simulink model "conSys_3robots_1_vR2014a"  (Simulink 8.3)
settings: Solver=ode3  StartTime=0.0  StopTime=200  FixedStep=Ts  RelTol=1e-3
values from neighbouring files (symbols this model uses):
  ck = double(max(abs([par.q0_r1;par.q0_r2] - [par.q0r_r1;par.q0r_r2]))*20/7000 + 6)    [startUp_conSys_2robots_1_vGPU_vR2014a.m]    (also in startUp_conSys_2robots_1_vR2014a.m = max(abs([par.q0_r1;par.q0_r2] - [par.q0r_r1;par.q0r_r2]))*20; startUp_conSys_2robots_2_vR2014a.m = max(abs([par.q0_r1;par.q0_r2] - [par.q0r_r1;par.q0r_r2]))*20; startUp_conSys_2robots_3_vR2014a.m = max(abs([par.q0_r1;par.q0_r2] - [par.q0r_r1;par.q0r_r2]))*20; startUp_conSys_2robots_4_vR2014a.m = max(abs([par.q0_r1;par.q0_r2] - [par.q0r_r1;par.q0r_r2]))*20)
  d0t = dt*ht    (= 0.328)    [startUp_conSys_2robots_1_vGPU_vR2014a.m]    (also in startUp_conSys_2robots_1_vR2014a.m; startUp_conSys_2robots_2_vR2014a.m; startUp_conSys_2robots_3_vR2014a.m; startUp_conSys_2robots_4_vR2014a.m)
  dt = rt*ht    (= 16.4)    [startUp_conSys_2robots_1_vGPU_vR2014a.m]    (also in startUp_conSys_2robots_1_vR2014a.m; startUp_conSys_2robots_2_vR2014a.m; startUp_conSys_2robots_3_vR2014a.m; startUp_conSys_2robots_4_vR2014a.m)
  dx1r_0 = dxc_0 + sin(thc_0)*dd_0 + d_0*cos(thc_0)*dthc_0    [startUp_conSys_2robots_1_vGPU_vR2014a.m]    (also in startUp_conSys_2robots_1_vR2014a.m; startUp_conSys_2robots_2_vR2014a.m; startUp_conSys_2robots_3_vR2014a.m; startUp_conSys_2robots_4_vR2014a.m)
  dx2r_0 = dxc_0 - sin(thc_0)*dd_0 - d_0*cos(thc_0)*dthc_0    [startUp_conSys_2robots_1_vGPU_vR2014a.m]    (also in startUp_conSys_2robots_1_vR2014a.m; startUp_conSys_2robots_2_vR2014a.m; startUp_conSys_2robots_3_vR2014a.m; startUp_conSys_2robots_4_vR2014a.m)
  dy1r_0 = dyc_0 + cos(thc_0)*dd_0 - d_0*sin(thc_0)*dthc_0    [startUp_conSys_2robots_1_vGPU_vR2014a.m]    (also in startUp_conSys_2robots_1_vR2014a.m; startUp_conSys_2robots_2_vR2014a.m; startUp_conSys_2robots_3_vR2014a.m; startUp_conSys_2robots_4_vR2014a.m)
  dy2r_0 = dyc_0 - cos(thc_0)*dd_0 + d_0*sin(thc_0)*dthc_0    [startUp_conSys_2robots_1_vGPU_vR2014a.m]    (also in startUp_conSys_2robots_1_vR2014a.m; startUp_conSys_2robots_2_vR2014a.m; startUp_conSys_2robots_3_vR2014a.m; startUp_conSys_2robots_4_vR2014a.m)
  ht = .02    (= 0.02)    [startUp_conSys_2robots_1_vGPU_vR2014a.m]    (also in startUp_conSys_2robots_1_vR2014a.m; startUp_conSys_2robots_2_vR2014a.m; startUp_conSys_2robots_3_vR2014a.m; startUp_conSys_2robots_4_vR2014a.m)
  rt = 820    [startUp_conSys_2robots_1_vGPU_vR2014a.m]    (also in startUp_conSys_2robots_1_vR2014a.m; startUp_conSys_2robots_2_vR2014a.m; startUp_conSys_2robots_3_vR2014a.m; startUp_conSys_2robots_4_vR2014a.m)
  TD = ss(Atd,Btd,Ctd,Dtd,Ts)    [startUp_conSys_2robots_1_vGPU_vR2014a.m]    (also in startUp_conSys_2robots_1_vR2014a.m; startUp_conSys_2robots_2_vR2014a.m; startUp_conSys_2robots_3_vR2014a.m; startUp_conSys_2robots_4_vR2014a.m)
  Ts = 1/200    (= 0.005)    [startUp_conSys_2robots_1_vGPU_vR2014a.m]    (also in startUp_conSys_2robots_1_vR2014a.m = 0.0125; startUp_conSys_2robots_2_vR2014a.m = 0.01; startUp_conSys_2robots_3_vR2014a.m; startUp_conSys_2robots_4_vR2014a.m)
undefined symbols (not defined in the file or in its folder): Beta_Correction_1b, Beta_Correction_2b, Beta_Correction_3b, Beta_Correction_4b, DiscIntNeverNeededParam, dth1r_0, dth2r_0, dth3r_0, dx3r_0, dy3r_0, par, th1r_0, th2r_0, th3r_0, x1r_0, x2r_0, x3r_0, y1r_0, y2r_0, y3r_0
undefined symbols (not defined in the file): ADAMS_cwd, ADAMS_exec, ADAMS_host, ADAMS_init, ADAMS_inputs, ADAMS_outputs, ADAMS_prefix, ADAMS_static, ADAMS_sysdir
libraries: simulink x26, cstblocks x11
(part 2 of 3)

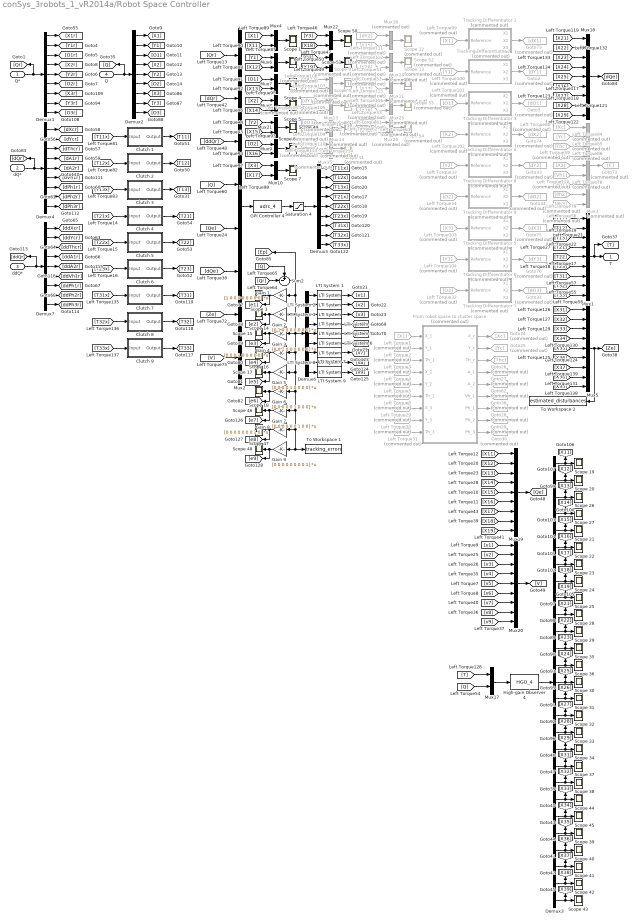
== system conSys_3robots_1_vR2014a/Robot Space Controller ==
  Q* : Inport
  dQ* : Inport  Port=2
  ddQ* : Inport  Port=3
  Q : Inport  Port=4
  Clutch 1 : Subsystem
  Clutch 2 : Subsystem
  Clutch 3 : Subsystem
  Clutch 4 : Subsystem
  Clutch 5 : Subsystem
  Clutch 6 : Subsystem
  Clutch 7 : Subsystem
  Clutch 8 : Subsystem
  Clutch 9 : Subsystem
  Demux{1..2,4..7} (6 alike) : Demux  Outputs=9
  Demux3 : Demux  Outputs=27
  From robot space to cluster space : Subsystem  Commented=on
  GPI Controller 4 : S-Function  FunctionName=adrc_4  Parameters=par  EnableBusSupport=off
  Gain 1 : Gain  Gain=[1 0 0 0 0 0 0 0 0]  Multiplication=Matrix(K*u)
  Gain 2 : Gain  Gain=[0 1 0 0 0 0 0 0 0]  Multiplication=Matrix(K*u)
  Gain 3 : Gain  Gain=[0 0 1 0 0 0 0 0 0]  Multiplication=Matrix(K*u)
  Gain 4 : Gain  Gain=[0 0 0 1 0 0 0 0 0]  Multiplication=Matrix(K*u)
  Gain 5 : Gain  Gain=[0 0 0 0 1 0 0 0 0]  Multiplication=Matrix(K*u)
  Gain 6 : Gain  Gain=[0 0 0 0 0 1 0 0 0]  Multiplication=Matrix(K*u)
  Gain 7 : Gain  Gain=[0 0 0 0 0 0 1 0 0]  Multiplication=Matrix(K*u)
  Gain 8 : Gain  Gain=[0 0 0 0 0 0 0 1 0]  Multiplication=Matrix(K*u)
  Gain 9 : Gain  Gain=[0 0 0 0 0 0 0 0 1]  Multiplication=Matrix(K*u)
  Goto2 : Goto  Commented=on  GotoTag=dY1
  Goto24 : Goto  Commented=on  GotoTag=Xc
  Goto25 : Goto  Commented=on  GotoTag=Yc
  Goto26 : Goto  Commented=on  GotoTag=Thc
  Goto27 : Goto  Commented=on  GotoTag=A1
  Goto28 : Goto  Commented=on  GotoTag=Ph1
  Goto29 : Goto  Commented=on  GotoTag=Ph2
  Goto3 : Goto  Commented=on  GotoTag=dO1
  Goto30 : Goto  Commented=on  GotoTag=Ph3
  Goto32 : Goto  Commented=on  GotoTag=dO3
  Goto33 : Goto  Commented=on  GotoTag=dY2
  Goto34 : Goto  Commented=on  GotoTag=dO2
  Goto36 : Goto  Commented=on  GotoTag=Vh1
  Goto62 : Goto  Commented=on  GotoTag=A2
  Goto72 : Goto  Commented=on  GotoTag=C
  Goto73 : Goto  Commented=on  GotoTag=dX1
  Goto74 : Goto  Commented=on  GotoTag=dX2
  Goto75 : Goto  Commented=on  GotoTag=dX3
  Goto76 : Goto  Commented=on  GotoTag=dY3
  High-gain Observer 4 : S-Function  FunctionName=HGO_4  Parameters=par  EnableBusSupport=off
  LTI System {1..2,4..5,7..8} (6 alike) : cstblocks/LTI System  sys=par.Gz_1  IC=[]
  LTI System 3 : cstblocks/LTI System  sys=par.Gz_2  IC=[]
  LTI System 6 : cstblocks/LTI System  sys=par.Gz_2  IC=[]
  LTI System 9 : cstblocks/LTI System  sys=par.Gz_2  IC=[]
  Left Torque1 : From  Commented=on  GotoTag=X1
  Left Torque100 : From  Commented=on  GotoTag=Y1
  Left Torque101 : From  Commented=on  GotoTag=O1
  Left Torque102 : From  Commented=on  GotoTag=X2
  Left Torque103 : From  Commented=on  GotoTag=X3
  Left Torque104 : From  Commented=on  GotoTag=Y3
  Left Torque105 : From  Commented=on  GotoTag=dY1
  Left Torque106 : From  Commented=on  GotoTag=X22
  Left Torque107 : From  Commented=on  GotoTag=dX1
  Left Torque108 : From  Commented=on  GotoTag=X21
  Left Torque109 : From  Commented=on  GotoTag=dO1
  Left Torque110 : From  Commented=on  GotoTag=X23
  Left Torque111 : From  Commented=on  GotoTag=dY2
  Left Torque112 : From  Commented=on  GotoTag=X25
  Left Torque113 : From  Commented=on  GotoTag=dX2
  Left Torque114 : From  Commented=on  GotoTag=X24
  Left Torque115 : From  Commented=on  GotoTag=dX3
  Left Torque116 : From  Commented=on  GotoTag=X27
  Left Torque120 : From  Commented=on  GotoTag=Vh1
  Left Torque2 : From  Commented=on  GotoTag=Y1
  Left Torque29 : From  Commented=on  GotoTag=X3
  Left Torque3 : From  Commented=on  GotoTag=O1
  Left Torque30 : From  Commented=on  GotoTag=Y3
  Left Torque31 : From  Commented=on  GotoTag=O3
  Left Torque32 : From  Commented=on  GotoTag=O3
  Left Torque33 : From  Commented=on  GotoTag=Y2
  Left Torque34 : From  Commented=on  GotoTag=O2
  Left Torque4 : From  Commented=on  GotoTag=X2
  Left Torque5 : From  Commented=on  GotoTag=Y2
  Left Torque51 : From  Commented=on  GotoTag=dO2
  Left Torque52 : From  Commented=on  GotoTag=X26
  Left Torque53 : From  Commented=on  GotoTag=dY3
  Left Torque58 : From  Commented=on  GotoTag=Ph3
  Left Torque59 : From  Commented=on  GotoTag=A2
  Left Torque6 : From  Commented=on  GotoTag=O2
  Left Torque61 : From  Commented=on  GotoTag=X28
  Left Torque62 : From  Commented=on  GotoTag=dO3
  Left Torque63 : From  Commented=on  GotoTag=X29
  Left Torque78 : From  Commented=on  GotoTag=Ph1
  Left Torque79 : From  Commented=on  GotoTag=Ph2
  Left Torque80 : From  Commented=on  GotoTag=Xc
  Left Torque84 : From  Commented=on  GotoTag=Yc
  Left Torque85 : From  Commented=on  GotoTag=Thc
  Left Torque86 : From  Commented=on  GotoTag=A1
  Left Torque99 : From  Commented=on  GotoTag=X1
  Mux{1,5,18..20} (5 alike) : Mux  Inputs=9
  Mux{4,6..10,17,21..23} (10 alike) : Mux  Inputs=2
  Mux{11..16,24..26} (9 alike) : Mux  Commented=on  Inputs=2
  Mux2 : Mux  Inputs=8
  Mux3 : Mux  Commented=on  Inputs=9
  Saturation 4 : Saturate  UpperLimit=100  LowerLimit=-100
  Scope {1..7,14..51} (45 alike) : Scope
      Scope 1 settings: YMin=-2000  YMax=16000  SaveName=ScopeData37
      Scope 14 settings: YMin=-100  YMax=2000  SaveName=ScopeData77
      Scope 15 settings: YMin=-1  YMax=4  SaveName=ScopeData78
      Scope 16 settings: YMin=-100  YMax=2000  SaveName=ScopeData82
      Scope 17 settings: YMin=-100  YMax=2000  SaveName=ScopeData83
      Scope 18 settings: YMin=-1  YMax=4  SaveName=ScopeData84
      Scope 19 settings: YMin=-2000  YMax=16000  SaveName=ScopeData86
      Scope 2 settings: YMin=-2000  YMax=16000  SaveName=ScopeData39
      Scope 20 settings: YMin=0  YMax=10000  SaveName=ScopeData87
      Scope 21 settings: YMin=0  YMax=5000  SaveName=ScopeData88
      Scope 22 settings: SaveName=ScopeData90
      Scope 23 settings: YMin=-10  YMax=100  SaveName=ScopeData91
      Scope 24 settings: YMin=-50  YMax=50  SaveName=ScopeData92
      Scope 25 settings: YMin=-6  YMax=6  SaveName=ScopeData93
      Scope 26 settings: SaveName=ScopeData94
      Scope 27 settings: TimeRange=388  YMin=-6  YMax=60  SaveName=ScopeData95
      Scope 28 settings: YMin=0  YMax=10000  SaveName=ScopeData96
      Scope 29 settings: YMin=0  YMax=10000  SaveName=ScopeData97
      Scope 3 settings: YMin=-100  YMax=2000  SaveName=ScopeData40
      Scope 30 settings: YMin=-50  YMax=50  SaveName=ScopeData98
      Scope 31 settings: YMin=-1  YMax=1  SaveName=ScopeData99
      Scope 32 settings: YMin=-60  YMax=60  SaveName=ScopeData100
      Scope 33 settings: YMin=-1  YMax=1  SaveName=ScopeData101
      Scope 34 settings: YMin=-1  YMax=1  SaveName=ScopeData102
      Scope 35 settings: SaveName=ScopeData103
      Scope 36 settings: YMin=-60  YMax=60  SaveName=ScopeData104
      Scope 37 settings: YMin=-600  YMax=600  SaveName=ScopeData26
      Scope 38 settings: YMin=-600  YMax=600  SaveName=ScopeData27
      Scope 39 settings: YMin=-600  YMax=600  SaveName=ScopeData28
      Scope 4 settings: YMin=-2000  YMax=16000  SaveName=ScopeData41
      Scope 40 settings: YMin=-1  YMax=1  SaveName=ScopeData42
      Scope 41 settings: YMin=-600  YMax=600  SaveName=ScopeData52
      Scope 42 settings: YMin=-600  YMax=600  SaveName=ScopeData53
      Scope 43 settings: YMin=-1  YMax=1  SaveName=ScopeData54
      Scope 44 settings: SaveName=ScopeData55
      Scope 45 settings: YMin=-600  YMax=600  SaveName=ScopeData56
      Scope 46 settings: YMin=-100  YMax=2000  SaveName=ScopeData57
      Scope 47 settings: YMin=-100  YMax=2000  SaveName=ScopeData58
      Scope 48 settings: YMin=-1  YMax=4  SaveName=ScopeData59
      Scope 49 settings: YMin=-2000  YMax=16000  SaveName=ScopeData60
      Scope 5 settings: YMin=-2000  YMax=16000  SaveName=ScopeData43
      Scope 50 settings: YMin=-20  YMax=20  SaveName=ScopeData62
      Scope 51 settings: YMin=-20  YMax=20  SaveName=ScopeData63
      Scope 6 settings: YMin=-20  YMax=20  SaveName=ScopeData44
      Scope 7 settings: YMin=-20  YMax=20  SaveName=ScopeData45
  Scope {8..13,52..54} (9 alike) : Scope  Commented=on
      Scope 10 settings: YMin=-2  YMax=2  SaveName=ScopeData46
      Scope 11 settings: YMin=-40  YMax=40  SaveName=ScopeData47
      Scope 12 settings: YMin=-2  YMax=2  SaveName=ScopeData73
      Scope 13 settings: YMin=-2  YMax=2  SaveName=ScopeData74
      Scope 52 settings: YMin=-2  YMax=2  SaveName=ScopeData64
      Scope 53 settings: YMin=-2  YMax=2  SaveName=ScopeData65
      Scope 54 settings: YMin=-2  YMax=2  SaveName=ScopeData66
      Scope 8 settings: YMin=-2000  YMax=16000  SaveName=ScopeData75
      Scope 9 settings: YMin=-2000  YMax=2000  SaveName=ScopeData76
  Sum2 : Sum  Inputs=+-|
  To Workspace 1 : ToWorkspace  VariableName=tracking_errors  SaveFormat=Structure With Time  SampleTime=-1
  To Workspace 2 : ToWorkspace  VariableName=estimated_disturbances  SaveFormat=Structure With Time  SampleTime=-1
  Tracking Differentiator 1 : Subsystem  Commented=on
  Tracking Differentiator 2 : Subsystem  Commented=on
  Tracking Differentiator 3 : Subsystem  Commented=on
  Tracking Differentiator 4 : Subsystem  Commented=on
  Tracking Differentiator 5 : Subsystem  Commented=on
  Tracking Differentiator 6 : Subsystem  Commented=on
  Tracking Differentiator 7 : Subsystem  Commented=on
  Tracking Differentiator 8 : Subsystem  Commented=on
  Tracking Differentiator 9 : Subsystem  Commented=on
  T : Outport
  wires:
  From robot space to cluster space/5(A_2) -> Goto62/1
  From robot space to cluster space/8(Ph_2) -> Goto29/1
  From robot space to cluster space/7(Ph_1) -> Goto28/1
  From robot space to cluster space/3(Th_c) -> Goto26/1
  From robot space to cluster space/2(Y_c) -> Goto25/1
  From robot space to cluster space/1(X_c) -> Goto24/1
  Q/1 -> Demux2/1, [Q]
  Demux2/1 -> [X1]
  Demux2/2 -> [Y1]
  Demux2/3 -> [O1]
  Demux2/4 -> [X2]
  Demux2/5 -> [Y2]
  Demux2/6 -> [O2]
  Left Torque1/1 -> From robot space to cluster space/1(X_1)
  Left Torque2/1 -> From robot space to cluster space/2(Y_1)
  Left Torque3/1 -> From robot space to cluster space/3(Th_1)
  Left Torque4/1 -> From robot space to cluster space/4(X_2)
  Left Torque5/1 -> From robot space to cluster space/5(Y_2)
  Left Torque6/1 -> From robot space to cluster space/6(Th_2)
  Mux2/1 -> GPI Controller 4/1
  Demux5/1 -> [T11x]
  Demux5/2 -> [T12x]
  Demux5/3 -> [T13x]
  GPI Controller 4/1 -> Saturation 4/1
  Saturation 4/1 -> Demux5/1
  Demux5/4 -> [T21x]
  Demux5/5 -> [T22x]
  Demux5/6 -> [T23x]
  [Qr] -> Sum2/2
  [Q] -> Sum2/1
  Demux6/1 -> LTI System 1/1
  Demux6/2 -> LTI System 2/1
  Demux6/3 -> LTI System 3/1
  [T11x] -> Clutch 1/1(Input)
  Clutch 1/1(Output) -> [T11]
  [T12x] -> Clutch 2/1(Input)
  Clutch 2/1(Output) -> [T12]
  [T13x] -> Clutch 3/1(Input)
  Clutch 3/1(Output) -> [T13]
  [T21x] -> Clutch 4/1(Input)
  Clutch 4/1(Output) -> [T21]
  [T22x] -> Clutch 5/1(Input)
  Clutch 5/1(Output) -> [T22]
  [T23x] -> Clutch 6/1(Input)
  Clutch 6/1(Output) -> [T23]
  [T11] -> Mux1/1
  [T23] -> Mux1/6
  [T21] -> Mux1/4
  [T22] -> Mux1/5
  [T12] -> Mux1/2
  [T13] -> Mux1/3
  Mux1/1 -> [T], T/1
  Q*/1 -> [Qr], Demux1/1
  Demux1/1 -> [X1r]
  Demux1/2 -> [Y1r]
  Demux1/3 -> [O1r]
  Demux1/4 -> [X2r]
  Demux1/5 -> [Y2r]
  Demux1/6 -> [O2r]
  dQ*/1 -> [dQr], Demux4/1
  Demux4/1 -> [dXcr]
  Demux4/2 -> [dYcr]
  Demux4/3 -> [dThcr]
  Demux4/4 -> [dA1r]
  Demux7/1 -> [ddXcr]
  Demux7/2 -> [ddYcr]
  Demux7/3 -> [ddThcr]
  Demux7/4 -> [ddA1r]
  ddQ*/1 -> [ddQr], Demux7/1
  Demux6/4 -> LTI System 4/1
  Demux6/5 -> LTI System 5/1
  Demux6/6 -> LTI System 6/1
  [Qr] -> Mux2/1
  [ddQr] -> Mux2/3
  [Q] -> Mux2/4
  [Ze] -> Mux2/7
  [Qe] -> Mux2/5
  [dQe] -> Mux2/6
  [V] -> Mux2/8
  Left Torque80/1 -> Mux3/1
  Left Torque86/1 -> Mux3/4
  Left Torque84/1 -> Mux3/2
  Left Torque85/1 -> Mux3/3
  Mux3/1 -> Goto72/1
  [X11] -> Mux4/2
  [X1] -> Mux4/1
  Mux4/1 -> Scope 1/1
  [X12] -> Mux6/2
  [Y1] -> Mux6/1
  Mux6/1 -> Scope 2/1
  [X13] -> Mux7/2
  [O1] -> Mux7/1
  Mux7/1 -> Scope 4/1
  [X14] -> Mux8/2
  [X2] -> Mux8/1
  Mux8/1 -> Scope 5/1
  [X16] -> Mux9/2
  [O2] -> Mux9/1
  Mux9/1 -> Scope 6/1
  [X17] -> Mux10/2
  [X3] -> Mux10/1
  Mux10/1 -> Scope 7/1
  Left Torque99/1 -> Tracking Differentiator 1/1(Reference)
  Left Torque100/1 -> Tracking Differentiator 2/1(Reference)
  Left Torque101/1 -> Tracking Differentiator 3/1(Reference)
  Left Torque102/1 -> Tracking Differentiator 4/1(Reference)
  Left Torque103/1 -> Tracking Differentiator 5/1(Reference)
  Left Torque104/1 -> Tracking Differentiator 6/1(Reference)
  Tracking Differentiator 1/2(X2) -> Goto73/1
  Tracking Differentiator 2/2(X2) -> Goto2/1
  Tracking Differentiator 3/2(X2) -> Goto3/1
  Tracking Differentiator 4/2(X2) -> Goto74/1
  Tracking Differentiator 5/2(X2) -> Goto75/1
  Tracking Differentiator 6/2(X2) -> Goto76/1
  Left Torque108/1 -> Mux12/2
  Left Torque107/1 -> Mux12/1
  Mux12/1 -> Scope 8/1
  Left Torque106/1 -> Mux13/2
  Left Torque105/1 -> Mux13/1
  Mux13/1 -> Scope 9/1
  Left Torque110/1 -> Mux14/2
  Left Torque109/1 -> Mux14/1
  Mux14/1 -> Scope 10/1
  Left Torque114/1 -> Mux15/2
  Left Torque113/1 -> Mux15/1
  Mux15/1 -> Scope 11/1
  Left Torque112/1 -> Mux16/2
  Left Torque111/1 -> Mux16/1
  Mux16/1 -> Scope 12/1
  Left Torque116/1 -> Mux11/2
  Left Torque115/1 -> Mux11/1
  Mux11/1 -> Scope 13/1
  LTI System 1/1 -> [v1]
  LTI System 2/1 -> [v2]
  LTI System 3/1 -> [v3]
  LTI System 4/1 -> [v4]
  LTI System 5/1 -> [v5]
  LTI System 6/1 -> [v6]
  Gain 1/1 -> [e1], Scope 3/1
  Gain 2/1 -> [e2], Scope 14/1
  Gain 3/1 -> [e3], Scope 15/1
  Gain 4/1 -> [e4], Scope 16/1
  Gain 5/1 -> [e5], Scope 17/1
  Gain 6/1 -> [e6], Scope 18/1
  Mux17/1 -> High-gain Observer 4/1
  Demux3/9 -> Scope 25/1, [X19]
  Demux3/7 -> [X17], Scope 23/1
  Demux3/8 -> [X18], Scope 24/1
  Demux3/5 -> [X15], Scope 21/1
  Demux3/6 -> [X16], Scope 22/1
  High-gain Observer 4/1 -> Demux3/1
  Demux3/3 -> Scope 26/1, [X13]
  Demux3/4 -> Scope 27/1, [X14]
  Demux3/1 -> Scope 19/1, [X11]
  Demux3/2 -> Scope 20/1, [X12]
  Demux3/17 -> Scope 33/1, [X28]
  Demux3/13 -> [X24], Scope 36/1
  Demux3/12 -> [X23], Scope 35/1
  Demux3/18 -> [X29], Scope 34/1
  Demux3/15 -> Scope 31/1, [X26]
  Demux3/10 -> [X21], Scope 28/1
  Demux3/11 -> [X22], Scope 29/1
  Demux3/16 -> Scope 32/1, [X27]
  Demux3/14 -> Scope 30/1, [X25]
  [X21] -> Mux18/1
  [X26] -> Mux18/6
  [X24] -> Mux18/4
  [X25] -> Mux18/5
  [X22] -> Mux18/2
  [X23] -> Mux18/3
  Mux18/1 -> [dQe]
  Demux2/7 -> [X3]
  Demux2/8 -> [Y3]
  Demux2/9 -> [O3]
  Demux1/7 -> [X3r]
  Demux1/8 -> [Y3r]
  Demux1/9 -> [O3r]
  Demux4/7 -> [dPh1r]
  Demux4/8 -> [dPh2r]
  Demux4/5 -> [dA2r]
  Demux4/6 -> [dVh1r]
  Demux4/9 -> [dPh3r]
  Demux7/7 -> [ddPh1r]
  Demux7/8 -> [ddPh2r]
  Demux7/9 -> [ddPh3r]
  Demux7/5 -> [ddA2r]
  Demux7/6 -> [ddVh1r]
  [T31x] -> Clutch 7/1(Input)
  Clutch 7/1(Output) -> [T31]
  [T32x] -> Clutch 8/1(Input)
  Clutch 8/1(Output) -> [T32]
  [T33x] -> Clutch 9/1(Input)
  Clutch 9/1(Output) -> [T33]
  Left Torque29/1 -> From robot space to cluster space/7(X_3)
  Left Torque30/1 -> From robot space to cluster space/8(Y_3)
  Left Torque31/1 -> From robot space to cluster space/9(Th_3)
  From robot space to cluster space/4(A_1) -> Goto27/1
  From robot space to cluster space/6(Vh_1) -> Goto36/1
  From robot space to cluster space/9(Ph_3) -> Goto30/1
  Left Torque32/1 -> Tracking Differentiator 7/1(Reference)
  Tracking Differentiator 7/2(X2) -> Goto32/1
  Left Torque33/1 -> Tracking Differentiator 8/1(Reference)
  Tracking Differentiator 8/2(X2) -> Goto33/1
  Left Torque34/1 -> Tracking Differentiator 9/1(Reference)
  Tracking Differentiator 9/2(X2) -> Goto34/1
  [T] -> Mux17/1
  [Q] -> Mux17/2
  [T33] -> Mux1/9
  [T31] -> Mux1/7
  [T32] -> Mux1/8
  Left Torque59/1 -> Mux3/5
  Left Torque58/1 -> Mux3/9
  Left Torque120/1 -> Mux3/6
  Left Torque78/1 -> Mux3/7
  Left Torque79/1 -> Mux3/8
  [X27] -> Mux18/7
  [X29] -> Mux18/9
  [X28] -> Mux18/8
  [X31] -> Mux5/1
  [X36] -> Mux5/6
  [X34] -> Mux5/4
  [X35] -> Mux5/5
  [X32] -> Mux5/2
  [X33] -> Mux5/3
  Mux5/1 -> To Workspace 2/1, [Ze]
  [X39] -> Mux5/9
  [X37] -> Mux5/7
  [X38] -> Mux5/8
  Demux3/26 -> [X38], Scope 42/1
  Demux3/22 -> Scope 45/1, [X34]
  Demux3/21 -> Scope 44/1, [X33]
  Demux3/27 -> Scope 43/1, [X39]
  Demux3/24 -> [X36], Scope 40/1
  Demux3/19 -> Scope 37/1, [X31]
  Demux3/20 -> Scope 38/1, [X32]
  Demux3/25 -> [X37], Scope 41/1
  Demux3/23 -> [X35], Scope 39/1
  [X11] -> Mux19/1
  [X16] -> Mux19/6
  [X14] -> Mux19/4
  [X15] -> Mux19/5
  [X12] -> Mux19/2
  [X13] -> Mux19/3
  Mux19/1 -> [Qe]
  [X19] -> Mux19/9
  [X17] -> Mux19/7
  [X18] -> Mux19/8
  [v1] -> Mux20/1
  [v6] -> Mux20/6
  [v4] -> Mux20/4
  [v5] -> Mux20/5
  [v2] -> Mux20/2
  [v3] -> Mux20/3
  Mux20/1 -> [V]
  [v9] -> Mux20/9
  [v7] -> Mux20/7
  [v8] -> Mux20/8
  [dQr] -> Mux2/2
  Demux5/7 -> [T31x]
  Demux5/8 -> [T32x]
  Demux5/9 -> [T33x]
  Demux6/7 -> LTI System 7/1
  LTI System 7/1 -> [v7]
  LTI System 8/1 -> [v8]
  LTI System 9/1 -> [v9]
  Demux6/8 -> LTI System 8/1
  Demux6/9 -> LTI System 9/1
  Gain 7/1 -> Scope 46/1, [e7]
  Gain 8/1 -> [e8], Scope 47/1
  Gain 9/1 -> Scope 48/1, [e9]
  [X15] -> Mux21/2
  Mux21/1 -> Scope 49/1
  [Y2] -> Mux21/1
  [X18] -> Mux22/2
  [Y3] -> Mux22/1
  Mux22/1 -> Scope 50/1
  [X19] -> Mux23/2
  [O3] -> Mux23/1
  Mux23/1 -> Scope 51/1
  Left Torque52/1 -> Mux24/2
  Left Torque51/1 -> Mux24/1
  Mux24/1 -> Scope 52/1
  Left Torque61/1 -> Mux25/2
  Left Torque53/1 -> Mux25/1
  Mux25/1 -> Scope 53/1
  Left Torque63/1 -> Mux26/2
  Left Torque62/1 -> Mux26/1
  Mux26/1 -> Scope 54/1
  Sum2/1 -> Demux6/1, To Workspace 1/1, Gain 9/1, Gain 8/1, Gain 7/1, Gain 6/1, Gain 5/1, Gain 4/1, Gain 3/1, Gain 2/1, Gain 1/1, [Ep]

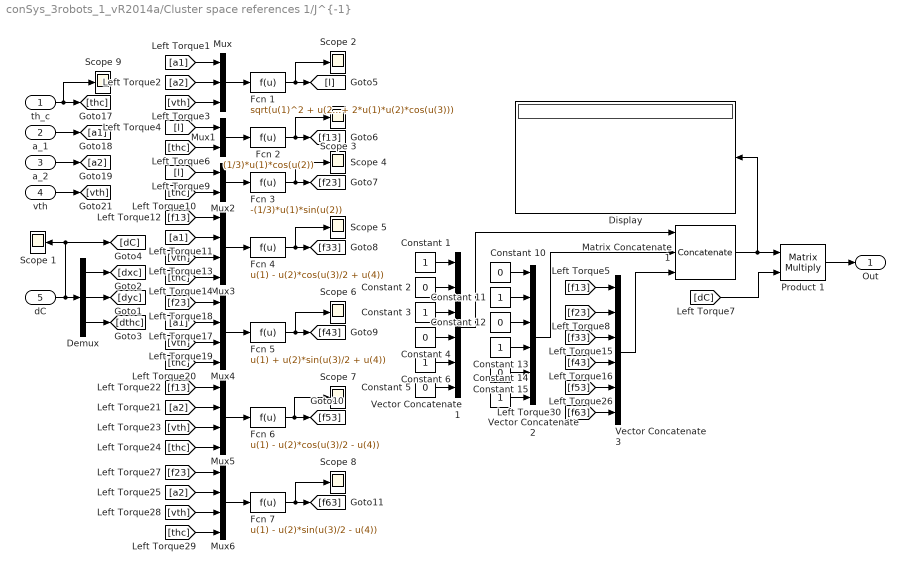
== system conSys_3robots_1_vR2014a/Cluster space references 1/J^{-1} ==
  th_c : Inport
  a_1 : Inport  Port=2
  a_2 : Inport  Port=3
  vth : Inport  Port=4
  dC : Inport  Port=5  PortDimensions=3
  Constant {1,3,6,11,13..14} (6 alike) : Constant
  Constant {2,4..5,10,12,15} (6 alike) : Constant  Value=0
  Demux : Demux  Outputs=3
  Display : Display
  Fcn 1 : Fcn  Expr=sqrt(u(1)^2 + u(2)^2 + 2*u(1)*u(2)*cos(u(3)))
  Fcn 2 : Fcn  Expr=(1/3)*u(1)*cos(u(2))
  Fcn 3 : Fcn  Expr=-(1/3)*u(1)*sin(u(2))
  Fcn 4 : Fcn  Expr=u(1) - u(2)*cos(u(3)/2 + u(4))
  Fcn 5 : Fcn  Expr=u(1) + u(2)*sin(u(3)/2 + u(4))
  Fcn 6 : Fcn  Expr=u(1) - u(2)*cos(u(3)/2 - u(4))
  Fcn 7 : Fcn  Expr=u(1) - u(2)*sin(u(3)/2 - u(4))
  Matrix Concatenate 1 : Concatenate  NumInputs=3  Mode=Multidimensional array  ConcatenateDimension=2
  Mux : Mux  Inputs=3
  Mux1 : Mux  Inputs=2
  Mux2 : Mux  Inputs=2
  Mux{3..6} (4 alike) : Mux
  Product 1 : Product  Multiplication=Matrix(*)
  Scope {1..9} (9 alike) : Scope
      Scope 1 settings: ShowLegends=on  YMin=-500  YMax=500  SaveName=ScopeData33
      Scope 2 settings: ShowLegends=on  YMin=-500  YMax=800  SaveName=ScopeData34
      Scope 3 settings: ShowLegends=on  YMin=-500  YMax=500  SaveName=ScopeData35
      Scope 4 settings: ShowLegends=on  YMin=-500  YMax=500  SaveName=ScopeData36
      Scope 5 settings: ShowLegends=on  YMin=-500  YMax=500  SaveName=ScopeData37
      Scope 6 settings: ShowLegends=on  YMin=-500  YMax=500  SaveName=ScopeData38
      Scope 7 settings: ShowLegends=on  YMin=-500  YMax=500  SaveName=ScopeData39
      Scope 8 settings: ShowLegends=on  YMin=-500  YMax=500  SaveName=ScopeData40
      Scope 9 settings: ShowLegends=on  YMin=-10  YMax=10  SaveName=ScopeData41
  Vector Concatenate 1 : Concatenate  NumInputs=6
  Vector Concatenate 2 : Concatenate  NumInputs=6
  Vector Concatenate 3 : Concatenate  NumInputs=6
  Out : Outport
  wires:
  [f53] -> Vector Concatenate 3/5
  [f43] -> Vector Concatenate 3/4
  [f23] -> Vector Concatenate 3/2
  [f13] -> Vector Concatenate 3/1
  Constant 14/1 -> Vector Concatenate 2/6
  Constant 15/1 -> Vector Concatenate 2/5
  Constant 13/1 -> Vector Concatenate 2/4
  Constant 12/1 -> Vector Concatenate 2/3
  Constant 11/1 -> Vector Concatenate 2/2
  Constant 10/1 -> Vector Concatenate 2/1
  Vector Concatenate 1/1 -> Matrix Concatenate 1/1
  Constant 5/1 -> Vector Concatenate 1/6
  Constant 6/1 -> Vector Concatenate 1/5
  Constant 4/1 -> Vector Concatenate 1/4
  Constant 3/1 -> Vector Concatenate 1/3
  Constant 2/1 -> Vector Concatenate 1/2
  Constant 1/1 -> Vector Concatenate 1/1
  vth/1 -> [vth]
  a_2/1 -> [a2]
  a_1/1 -> [a1]
  th_c/1 -> Scope 9/1, [thc]
  dC/1 -> Scope 1/1, [dC], Demux/1
  Demux/1 -> [dxc]
  Demux/2 -> [dyc]
  Demux/3 -> [dthc]
  [vth] -> Mux/3
  [a1] -> Mux/1
  [a2] -> Mux/2
  Mux/1 -> Fcn 1/1
  Fcn 1/1 -> Scope 2/1, [l]
  [l] -> Mux1/1
  [thc] -> Mux1/2
  Mux1/1 -> Fcn 2/1
  Fcn 2/1 -> Scope 3/1, [f13]
  Vector Concatenate 2/1 -> Matrix Concatenate 1/2
  Vector Concatenate 3/1 -> Matrix Concatenate 1/3
  Matrix Concatenate 1/1 -> Product 1/1, Display/1
  [dC] -> Product 1/2
  Product 1/1 -> Out/1
  [l] -> Mux2/1
  [thc] -> Mux2/2
  Mux2/1 -> Fcn 3/1
  Fcn 3/1 -> Scope 4/1, [f23]
  [f13] -> Mux3/1
  [a1] -> Mux3/2
  Mux3/1 -> Fcn 4/1
  Fcn 4/1 -> Scope 5/1, [f33]
  [vth] -> Mux3/3
  [thc] -> Mux3/4
  [f33] -> Vector Concatenate 3/3
  [f23] -> Mux4/1
  [a1] -> Mux4/2
  Mux4/1 -> Fcn 5/1
  Fcn 5/1 -> Scope 6/1, [f43]
  [vth] -> Mux4/3
  [thc] -> Mux4/4
  [f13] -> Mux5/1
  [a2] -> Mux5/2
  Mux5/1 -> Fcn 6/1
  Fcn 6/1 -> Scope 7/1, [f53]
  [vth] -> Mux5/3
  [thc] -> Mux5/4
  [f23] -> Mux6/1
  [a2] -> Mux6/2
  Mux6/1 -> Fcn 7/1
  Fcn 7/1 -> Scope 8/1, [f63]
  [vth] -> Mux6/3
  [thc] -> Mux6/4
  [f63] -> Vector Concatenate 3/6

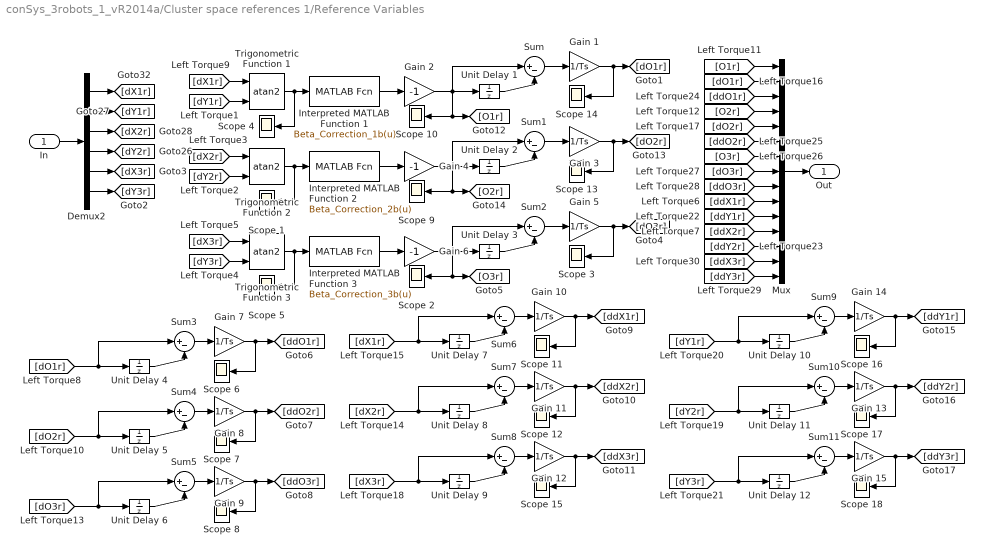
== system conSys_3robots_1_vR2014a/Cluster space references 1/Reference Variables ==
  In : Inport  PortDimensions=6
  Demux2 : Demux  Outputs=6
  Gain {1,3,5,7..15} (12 alike) : Gain  Gain=1/Ts
  Gain 2 : Gain  Gain=-1
  Gain 4 : Gain  Gain=-1
  Gain 6 : Gain  Gain=-1
  Interpreted MATLAB Function 1 : MATLABFcn  MATLABFcn=Beta_Correction_1b(u)  SampleTime=Ts
  Interpreted MATLAB Function 2 : MATLABFcn  MATLABFcn=Beta_Correction_2b(u)  SampleTime=Ts
  Interpreted MATLAB Function 3 : MATLABFcn  MATLABFcn=Beta_Correction_3b(u)  SampleTime=Ts
  Mux : Mux  Inputs=15
  Scope {1..18} (18 alike) : Scope
      Scope 1 settings: YMin=0  YMax=10  SaveName=ScopeData61
      Scope 10 settings: YMin=-10  YMax=0  SaveName=ScopeData68
      Scope 11 settings: YMin=-0.02  YMax=0.02  SaveName=ScopeData80
      Scope 12 settings: YMin=-0.45  YMax=0.47  SaveName=ScopeData81
      Scope 13 settings: YMin=-0.45  YMax=0.47  SaveName=ScopeData71
      Scope 14 settings: YMin=-0.45  YMax=0.47  SaveName=ScopeData72
      Scope 15 settings: YMin=-0.45  YMax=0.47  SaveName=ScopeData85
      Scope 16 settings: YMin=-0.02  YMax=0.02  SaveName=ScopeData105
      Scope 17 settings: YMin=-0.45  YMax=0.47  SaveName=ScopeData106
      Scope 18 settings: YMin=-0.45  YMax=0.47  SaveName=ScopeData107
      Scope 2 settings: YMin=-10  YMax=0  SaveName=ScopeData22
      Scope 3 settings: YMin=-0.45  YMax=0.47  SaveName=ScopeData29
      Scope 4 settings: YMin=0  YMax=10  SaveName=ScopeData30
      Scope 5 settings: YMin=0  YMax=10  SaveName=ScopeData31
      Scope 6 settings: YMin=-0.02  YMax=0.02  SaveName=ScopeData69
      Scope 7 settings: YMin=-0.45  YMax=0.47  SaveName=ScopeData70
      Scope 8 settings: YMin=-0.45  YMax=0.47  SaveName=ScopeData79
      Scope 9 settings: YMin=-10  YMax=0  SaveName=ScopeData67
  Sum{,1..11} (12 alike) : Sum  Inputs=|+-
  Trigonometric Function 1 : Trigonometry  Operator=atan2  SampleTime=Ts
  Trigonometric Function 2 : Trigonometry  Operator=atan2  SampleTime=Ts
  Trigonometric Function 3 : Trigonometry  Operator=atan2  SampleTime=Ts
  Unit Delay 1 : UnitDelay  InitialCondition=th1r_0  SampleTime=-1
  Unit Delay 10 : UnitDelay  InitialCondition=dy1r_0  SampleTime=-1
  Unit Delay 11 : UnitDelay  InitialCondition=dy2r_0  SampleTime=-1
  Unit Delay 12 : UnitDelay  InitialCondition=dy3r_0  SampleTime=-1
  Unit Delay 2 : UnitDelay  InitialCondition=th2r_0  SampleTime=-1
  Unit Delay 3 : UnitDelay  InitialCondition=th3r_0  SampleTime=-1
  Unit Delay 4 : UnitDelay  InitialCondition=dth1r_0  SampleTime=-1
  Unit Delay 5 : UnitDelay  InitialCondition=dth2r_0  SampleTime=-1
  Unit Delay 6 : UnitDelay  InitialCondition=dth3r_0  SampleTime=-1
  Unit Delay 7 : UnitDelay  InitialCondition=dx1r_0  SampleTime=-1
  Unit Delay 8 : UnitDelay  InitialCondition=dx2r_0  SampleTime=-1
  Unit Delay 9 : UnitDelay  InitialCondition=dx3r_0  SampleTime=-1
  Out : Outport  PortDimensions=15
  wires:
  In/1 -> Demux2/1
  Demux2/1 -> [dX1r]
  Demux2/2 -> [dY1r]
  Demux2/3 -> [dX2r]
  Demux2/4 -> [dY2r]
  [dX1r] -> Trigonometric Function 1/1
  [dY1r] -> Trigonometric Function 1/2
  Interpreted MATLAB Function 1/1 -> Gain 2/1
  Unit Delay 1/1 -> Sum/2
  Sum/1 -> Gain 1/1
  Gain 1/1 -> Scope 14/1, [dO1r]
  Trigonometric Function 1/1 -> Scope 4/1, Interpreted MATLAB Function 1/1
  Gain 2/1 -> Scope 10/1, [O1r], Sum/1, Unit Delay 1/1
  [dX2r] -> Trigonometric Function 2/1
  [dY2r] -> Trigonometric Function 2/2
  Interpreted MATLAB Function 2/1 -> Gain 4/1
  Unit Delay 2/1 -> Sum1/2
  Sum1/1 -> Gain 3/1
  Gain 3/1 -> Scope 13/1, [dO2r]
  Trigonometric Function 2/1 -> Scope 1/1, Interpreted MATLAB Function 2/1
  Gain 4/1 -> Unit Delay 2/1, Sum1/1, Scope 9/1, [O2r]
  Demux2/5 -> [dX3r]
  Demux2/6 -> [dY3r]
  [dX3r] -> Trigonometric Function 3/1
  [dY3r] -> Trigonometric Function 3/2
  Interpreted MATLAB Function 3/1 -> Gain 6/1
  Unit Delay 3/1 -> Sum2/2
  Sum2/1 -> Gain 5/1
  Gain 5/1 -> [dO3r], Scope 3/1
  Trigonometric Function 3/1 -> Scope 5/1, Interpreted MATLAB Function 3/1
  Gain 6/1 -> Unit Delay 3/1, Sum2/1, [O3r], Scope 2/1
  Unit Delay 4/1 -> Sum3/2
  Sum3/1 -> Gain 7/1
  Gain 7/1 -> Scope 6/1, [ddO1r]
  Unit Delay 5/1 -> Sum4/2
  Sum4/1 -> Gain 8/1
  Gain 8/1 -> [ddO2r], Scope 7/1
  [dO1r] -> Sum3/1, Unit Delay 4/1
  [dO2r] -> Unit Delay 5/1, Sum4/1
  Unit Delay 6/1 -> Sum5/2
  Sum5/1 -> Gain 9/1
  Gain 9/1 -> Scope 8/1, [ddO3r]
  [dO3r] -> Sum5/1, Unit Delay 6/1
  Unit Delay 7/1 -> Sum6/2
  Sum6/1 -> Gain 10/1
  Gain 10/1 -> [ddX1r], Scope 11/1
  Unit Delay 8/1 -> Sum7/2
  Sum7/1 -> Gain 11/1
  Gain 11/1 -> Scope 12/1, [ddX2r]
  [dX1r] -> Unit Delay 7/1, Sum6/1
  [dX2r] -> Sum7/1, Unit Delay 8/1
  Unit Delay 9/1 -> Sum8/2
  Sum8/1 -> Gain 12/1
  Gain 12/1 -> [ddX3r], Scope 15/1
  [dX3r] -> Unit Delay 9/1, Sum8/1
  Unit Delay 10/1 -> Sum9/2
  Sum9/1 -> Gain 14/1
  Gain 14/1 -> Scope 16/1, [ddY1r]
  Unit Delay 11/1 -> Sum10/2
  Sum10/1 -> Gain 13/1
  Gain 13/1 -> [ddY2r], Scope 17/1
  [dY1r] -> Sum9/1, Unit Delay 10/1
  [dY2r] -> Unit Delay 11/1, Sum10/1
  Unit Delay 12/1 -> Sum11/2
  Sum11/1 -> Gain 15/1
  Gain 15/1 -> Scope 18/1, [ddY3r]
  [dY3r] -> Sum11/1, Unit Delay 12/1
  Mux/1 -> Out/1
  [O1r] -> Mux/1
  [dO1r] -> Mux/2
  [dO2r] -> Mux/5
  [O2r] -> Mux/4
  [ddO1r] -> Mux/3
  [ddO2r] -> Mux/6
  [O3r] -> Mux/7
  [dO3r] -> Mux/8
  [ddO3r] -> Mux/9
  [ddX1r] -> Mux/10
  [ddX2r] -> Mux/12
  [ddY1r] -> Mux/11
  [ddY2r] -> Mux/13
  [ddY3r] -> Mux/15
  [ddX3r] -> Mux/14

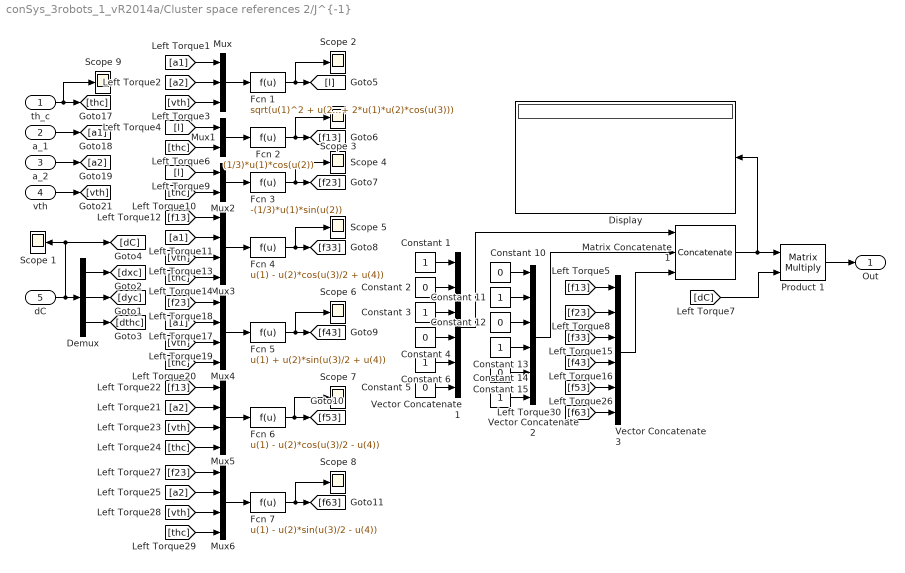
== system conSys_3robots_1_vR2014a/Cluster space references 2/J^{-1} ==
  th_c : Inport
  a_1 : Inport  Port=2
  a_2 : Inport  Port=3
  vth : Inport  Port=4
  dC : Inport  Port=5  PortDimensions=3
  Constant {1,3,6,11,13..14} (6 alike) : Constant
  Constant {2,4..5,10,12,15} (6 alike) : Constant  Value=0
  Demux : Demux  Outputs=3
  Display : Display
  Fcn 1 : Fcn  Expr=sqrt(u(1)^2 + u(2)^2 + 2*u(1)*u(2)*cos(u(3)))
  Fcn 2 : Fcn  Expr=(1/3)*u(1)*cos(u(2))
  Fcn 3 : Fcn  Expr=-(1/3)*u(1)*sin(u(2))
  Fcn 4 : Fcn  Expr=u(1) - u(2)*cos(u(3)/2 + u(4))
  Fcn 5 : Fcn  Expr=u(1) + u(2)*sin(u(3)/2 + u(4))
  Fcn 6 : Fcn  Expr=u(1) - u(2)*cos(u(3)/2 - u(4))
  Fcn 7 : Fcn  Expr=u(1) - u(2)*sin(u(3)/2 - u(4))
  Matrix Concatenate 1 : Concatenate  NumInputs=3  Mode=Multidimensional array  ConcatenateDimension=2
  Mux : Mux  Inputs=3
  Mux1 : Mux  Inputs=2
  Mux2 : Mux  Inputs=2
  Mux{3..6} (4 alike) : Mux
  Product 1 : Product  Multiplication=Matrix(*)
  Scope {1..9} (9 alike) : Scope
      Scope 1 settings: ShowLegends=on  YMin=-500  YMax=500  SaveName=ScopeData33
      Scope 2 settings: ShowLegends=on  YMin=-500  YMax=800  SaveName=ScopeData34
      Scope 3 settings: ShowLegends=on  YMin=-500  YMax=500  SaveName=ScopeData35
      Scope 4 settings: ShowLegends=on  YMin=-500  YMax=500  SaveName=ScopeData36
      Scope 5 settings: ShowLegends=on  YMin=-500  YMax=500  SaveName=ScopeData37
      Scope 6 settings: ShowLegends=on  YMin=-500  YMax=500  SaveName=ScopeData38
      Scope 7 settings: ShowLegends=on  YMin=-500  YMax=500  SaveName=ScopeData39
      Scope 8 settings: ShowLegends=on  YMin=-500  YMax=500  SaveName=ScopeData40
      Scope 9 settings: ShowLegends=on  YMin=-10  YMax=10  SaveName=ScopeData41
  Vector Concatenate 1 : Concatenate  NumInputs=6
  Vector Concatenate 2 : Concatenate  NumInputs=6
  Vector Concatenate 3 : Concatenate  NumInputs=6
  Out : Outport
  wires:
  [f63] -> Vector Concatenate 3/6
  [thc] -> Mux6/4
  [vth] -> Mux6/3
  Fcn 7/1 -> [f63], Scope 8/1
  Mux6/1 -> Fcn 7/1
  [a2] -> Mux6/2
  [f23] -> Mux6/1
  [thc] -> Mux5/4
  [vth] -> Mux5/3
  Fcn 6/1 -> [f53], Scope 7/1
  Mux5/1 -> Fcn 6/1
  [a2] -> Mux5/2
  [f13] -> Mux5/1
  [thc] -> Mux4/4
  [vth] -> Mux4/3
  Fcn 5/1 -> [f43], Scope 6/1
  Mux4/1 -> Fcn 5/1
  [a1] -> Mux4/2
  [f23] -> Mux4/1
  [f33] -> Vector Concatenate 3/3
  [thc] -> Mux3/4
  [vth] -> Mux3/3
  Fcn 4/1 -> [f33], Scope 5/1
  Mux3/1 -> Fcn 4/1
  [a1] -> Mux3/2
  [f13] -> Mux3/1
  Fcn 3/1 -> [f23], Scope 4/1
  Mux2/1 -> Fcn 3/1
  [thc] -> Mux2/2
  [l] -> Mux2/1
  Product 1/1 -> Out/1
  [dC] -> Product 1/2
  Matrix Concatenate 1/1 -> Display/1, Product 1/1
  Vector Concatenate 3/1 -> Matrix Concatenate 1/3
  Vector Concatenate 2/1 -> Matrix Concatenate 1/2
  Fcn 2/1 -> [f13], Scope 3/1
  Mux1/1 -> Fcn 2/1
  [thc] -> Mux1/2
  [l] -> Mux1/1
  Fcn 1/1 -> [l], Scope 2/1
  Mux/1 -> Fcn 1/1
  [a2] -> Mux/2
  [a1] -> Mux/1
  [vth] -> Mux/3
  Demux/3 -> [dthc]
  Demux/2 -> [dyc]
  Demux/1 -> [dxc]
  dC/1 -> Demux/1, [dC], Scope 1/1
  th_c/1 -> [thc], Scope 9/1
  a_1/1 -> [a1]
  a_2/1 -> [a2]
  vth/1 -> [vth]
  Constant 1/1 -> Vector Concatenate 1/1
  Constant 2/1 -> Vector Concatenate 1/2
  Constant 3/1 -> Vector Concatenate 1/3
  Constant 4/1 -> Vector Concatenate 1/4
  Constant 6/1 -> Vector Concatenate 1/5
  Constant 5/1 -> Vector Concatenate 1/6
  Vector Concatenate 1/1 -> Matrix Concatenate 1/1
  Constant 10/1 -> Vector Concatenate 2/1
  Constant 11/1 -> Vector Concatenate 2/2
  Constant 12/1 -> Vector Concatenate 2/3
  Constant 13/1 -> Vector Concatenate 2/4
  Constant 15/1 -> Vector Concatenate 2/5
  Constant 14/1 -> Vector Concatenate 2/6
  [f13] -> Vector Concatenate 3/1
  [f23] -> Vector Concatenate 3/2
  [f43] -> Vector Concatenate 3/4
  [f53] -> Vector Concatenate 3/5

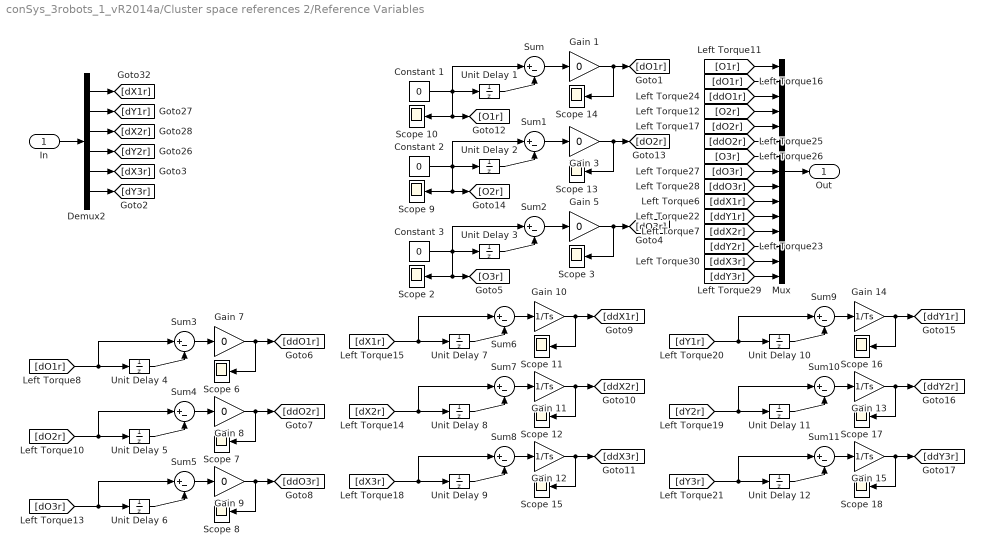
== system conSys_3robots_1_vR2014a/Cluster space references 2/Reference Variables ==
  In : Inport  PortDimensions=6
  Constant 1 : Constant  Value=0
  Constant 2 : Constant  Value=0
  Constant 3 : Constant  Value=0
  Demux2 : Demux  Outputs=6
  Gain {1,3,5,7..9} (6 alike) : Gain  Gain=0
  Gain {10..15} (6 alike) : Gain  Gain=1/Ts
  Mux : Mux  Inputs=15
  Scope {2..3,6..18} (15 alike) : Scope
      Scope 10 settings: YMin=-10  YMax=0  SaveName=ScopeData68
      Scope 11 settings: YMin=-0.02  YMax=0.02  SaveName=ScopeData80
      Scope 12 settings: YMin=-0.45  YMax=0.47  SaveName=ScopeData81
      Scope 13 settings: YMin=-0.45  YMax=0.47  SaveName=ScopeData71
      Scope 14 settings: YMin=-0.45  YMax=0.47  SaveName=ScopeData72
      Scope 15 settings: YMin=-0.45  YMax=0.47  SaveName=ScopeData85
      Scope 16 settings: YMin=-0.02  YMax=0.02  SaveName=ScopeData105
      Scope 17 settings: YMin=-0.45  YMax=0.47  SaveName=ScopeData106
      Scope 18 settings: YMin=-0.45  YMax=0.47  SaveName=ScopeData107
      Scope 2 settings: YMin=-10  YMax=0  SaveName=ScopeData22
      Scope 3 settings: YMin=-0.45  YMax=0.47  SaveName=ScopeData29
      Scope 6 settings: YMin=-0.02  YMax=0.02  SaveName=ScopeData69
      Scope 7 settings: YMin=-0.45  YMax=0.47  SaveName=ScopeData70
      Scope 8 settings: YMin=-0.45  YMax=0.47  SaveName=ScopeData79
      Scope 9 settings: YMin=-10  YMax=0  SaveName=ScopeData67
  Sum{,1..11} (12 alike) : Sum  Inputs=|+-
  Unit Delay 1 : UnitDelay  InitialCondition=th1r_0  SampleTime=-1
  Unit Delay 10 : UnitDelay  InitialCondition=dy1r_0  SampleTime=-1
  Unit Delay 11 : UnitDelay  InitialCondition=dy2r_0  SampleTime=-1
  Unit Delay 12 : UnitDelay  InitialCondition=dy3r_0  SampleTime=-1
  Unit Delay 2 : UnitDelay  InitialCondition=th2r_0  SampleTime=-1
  Unit Delay 3 : UnitDelay  InitialCondition=th3r_0  SampleTime=-1
  Unit Delay 4 : UnitDelay  InitialCondition=dth1r_0  SampleTime=-1
  Unit Delay 5 : UnitDelay  InitialCondition=dth2r_0  SampleTime=-1
  Unit Delay 6 : UnitDelay  InitialCondition=dth3r_0  SampleTime=-1
  Unit Delay 7 : UnitDelay  InitialCondition=dx1r_0  SampleTime=-1
  Unit Delay 8 : UnitDelay  InitialCondition=dx2r_0  SampleTime=-1
  Unit Delay 9 : UnitDelay  InitialCondition=dx3r_0  SampleTime=-1
  Out : Outport  PortDimensions=15
  wires:
  [ddX3r] -> Mux/14
  [ddY3r] -> Mux/15
  [ddY2r] -> Mux/13
  [ddY1r] -> Mux/11
  [ddX2r] -> Mux/12
  [ddX1r] -> Mux/10
  [ddO3r] -> Mux/9
  [dO3r] -> Mux/8
  [O3r] -> Mux/7
  [ddO2r] -> Mux/6
  [ddO1r] -> Mux/3
  [O2r] -> Mux/4
  [dO2r] -> Mux/5
  [dO1r] -> Mux/2
  [O1r] -> Mux/1
  Mux/1 -> Out/1
  [dY3r] -> Unit Delay 12/1, Sum11/1
  Gain 15/1 -> [ddY3r], Scope 18/1
  Sum11/1 -> Gain 15/1
  Unit Delay 12/1 -> Sum11/2
  [dY2r] -> Sum10/1, Unit Delay 11/1
  [dY1r] -> Unit Delay 10/1, Sum9/1
  Gain 13/1 -> Scope 17/1, [ddY2r]
  Sum10/1 -> Gain 13/1
  Unit Delay 11/1 -> Sum10/2
  Gain 14/1 -> [ddY1r], Scope 16/1
  Sum9/1 -> Gain 14/1
  Unit Delay 10/1 -> Sum9/2
  [dX3r] -> Sum8/1, Unit Delay 9/1
  Gain 12/1 -> Scope 15/1, [ddX3r]
  Sum8/1 -> Gain 12/1
  Unit Delay 9/1 -> Sum8/2
  [dX2r] -> Unit Delay 8/1, Sum7/1
  [dX1r] -> Sum6/1, Unit Delay 7/1
  Gain 11/1 -> [ddX2r], Scope 12/1
  Sum7/1 -> Gain 11/1
  Unit Delay 8/1 -> Sum7/2
  Gain 10/1 -> Scope 11/1, [ddX1r]
  Sum6/1 -> Gain 10/1
  Unit Delay 7/1 -> Sum6/2
  [dO3r] -> Unit Delay 6/1, Sum5/1
  Gain 9/1 -> [ddO3r], Scope 8/1
  Sum5/1 -> Gain 9/1
  Unit Delay 6/1 -> Sum5/2
  [dO2r] -> Sum4/1, Unit Delay 5/1
  [dO1r] -> Unit Delay 4/1, Sum3/1
  Gain 8/1 -> Scope 7/1, [ddO2r]
  Sum4/1 -> Gain 8/1
  Unit Delay 5/1 -> Sum4/2
  Gain 7/1 -> [ddO1r], Scope 6/1
  Sum3/1 -> Gain 7/1
  Unit Delay 4/1 -> Sum3/2
  Constant 3/1 -> Scope 2/1, [O3r], Sum2/1, Unit Delay 3/1
  Gain 5/1 -> Scope 3/1, [dO3r]
  Sum2/1 -> Gain 5/1
  Unit Delay 3/1 -> Sum2/2
  Demux2/6 -> [dY3r]
  Demux2/5 -> [dX3r]
  Constant 2/1 -> [O2r], Scope 9/1, Sum1/1, Unit Delay 2/1
  Gain 3/1 -> [dO2r], Scope 13/1
  Sum1/1 -> Gain 3/1
  Unit Delay 2/1 -> Sum1/2
  Constant 1/1 -> Unit Delay 1/1, Sum/1, [O1r], Scope 10/1
  Gain 1/1 -> [dO1r], Scope 14/1
  Sum/1 -> Gain 1/1
  Unit Delay 1/1 -> Sum/2
  Demux2/4 -> [dY2r]
  Demux2/3 -> [dX2r]
  Demux2/2 -> [dY1r]
  Demux2/1 -> [dX1r]
  In/1 -> Demux2/1

== system conSys_3robots_1_vR2014a/Omni Three-Robot ADAMS Model v2015/ADAMS Plant ==
  ADAMS inputs : Inport
  S-Function : S-Function  StopFcn=clear mex  FunctionName=adams_plant  Parameters=exevie,exesol,stat,outfil,nampre,o_rate,nam_in,namout,dft,modsim,modani,dt_out,inicmd,exetyp,comtyp,ada_host, workdir,pin_interp_order,pout_extrap_order,pin_extrap_order,pout_interp_order,simulink_lead_cosim  EnableBusSupport=off
  ADAMS outputs : Outport  InitialOutput=0
  wires:
  S-Function/1 -> ADAMS outputs/1
  ADAMS inputs/1 -> S-Function/1

== system conSys_3robots_1_vR2014a/Robot Space Controller/Clutch 1 ==
  Input : Inport
  Constant1 : Constant  Value=2
  Digital Clock : DigitalClock  SampleTime=Ts
  Gain 1 : Gain  Gain=.5
  Product : Product
  Rear Wheel Angular Speed5 : Scope
      settings: YMin=0  YMax=2  SaveName=ScopeData5
  Sine Wave1 : Sin  Bias=1  Frequency=(pi/ck)  Phase=-pi/2  SampleTime=Ts
  Switch : Switch  Threshold=ck
  Output : Outport
  wires:
  Constant1/1 -> Switch/1
  Digital Clock/1 -> Switch/2
  Switch/1 -> Gain 1/1
  Input/1 -> Product/2
  Product/1 -> Output/1
  Sine Wave1/1 -> Switch/3
  Gain 1/1 -> Rear Wheel Angular Speed5/1, Product/1

== system conSys_3robots_1_vR2014a/Robot Space Controller/Clutch 2 ==
  Input : Inport
  Constant1 : Constant  Value=2
  Digital Clock : DigitalClock  SampleTime=Ts
  Gain 1 : Gain  Gain=.5
  Product : Product
  Rear Wheel Angular Speed5 : Scope
      settings: YMin=0  YMax=2  SaveName=ScopeData5
  Sine Wave1 : Sin  Bias=1  Frequency=(pi/ck)  Phase=-pi/2  SampleTime=Ts
  Switch : Switch  Threshold=ck
  Output : Outport
  wires:
  Gain 1/1 -> Product/1, Rear Wheel Angular Speed5/1
  Sine Wave1/1 -> Switch/3
  Product/1 -> Output/1
  Input/1 -> Product/2
  Switch/1 -> Gain 1/1
  Digital Clock/1 -> Switch/2
  Constant1/1 -> Switch/1

== system conSys_3robots_1_vR2014a/Robot Space Controller/Clutch 3 ==
  Input : Inport
  Constant1 : Constant  Value=2
  Digital Clock : DigitalClock  SampleTime=Ts
  Gain 1 : Gain  Gain=.5
  Product : Product
  Rear Wheel Angular Speed5 : Scope
      settings: YMin=0  YMax=2  SaveName=ScopeData5
  Sine Wave1 : Sin  Bias=1  Frequency=(pi/ck)  Phase=-pi/2  SampleTime=Ts
  Switch : Switch  Threshold=ck
  Output : Outport
  wires:
  Constant1/1 -> Switch/1
  Digital Clock/1 -> Switch/2
  Switch/1 -> Gain 1/1
  Input/1 -> Product/2
  Product/1 -> Output/1
  Sine Wave1/1 -> Switch/3
  Gain 1/1 -> Rear Wheel Angular Speed5/1, Product/1

== system conSys_3robots_1_vR2014a/Robot Space Controller/Clutch 4 ==
  Input : Inport
  Constant1 : Constant  Value=2
  Digital Clock : DigitalClock  SampleTime=Ts
  Gain 1 : Gain  Gain=.5
  Product : Product
  Rear Wheel Angular Speed5 : Scope
      settings: YMin=0  YMax=2  SaveName=ScopeData5
  Sine Wave1 : Sin  Bias=1  Frequency=(pi/ck)  Phase=-pi/2  SampleTime=Ts
  Switch : Switch  Threshold=ck
  Output : Outport
  wires:
  Gain 1/1 -> Product/1, Rear Wheel Angular Speed5/1
  Sine Wave1/1 -> Switch/3
  Product/1 -> Output/1
  Input/1 -> Product/2
  Switch/1 -> Gain 1/1
  Digital Clock/1 -> Switch/2
  Constant1/1 -> Switch/1

== system conSys_3robots_1_vR2014a/Robot Space Controller/Clutch 5 ==
  Input : Inport
  Constant1 : Constant  Value=2
  Digital Clock : DigitalClock  SampleTime=Ts
  Gain 1 : Gain  Gain=.5
  Product : Product
  Rear Wheel Angular Speed5 : Scope
      settings: YMin=0  YMax=2  SaveName=ScopeData5
  Sine Wave1 : Sin  Bias=1  Frequency=(pi/ck)  Phase=-pi/2  SampleTime=Ts
  Switch : Switch  Threshold=ck
  Output : Outport
  wires:
  Constant1/1 -> Switch/1
  Digital Clock/1 -> Switch/2
  Switch/1 -> Gain 1/1
  Input/1 -> Product/2
  Product/1 -> Output/1
  Sine Wave1/1 -> Switch/3
  Gain 1/1 -> Rear Wheel Angular Speed5/1, Product/1

== system conSys_3robots_1_vR2014a/Robot Space Controller/Clutch 6 ==
  Input : Inport
  Constant1 : Constant  Value=2
  Digital Clock : DigitalClock  SampleTime=Ts
  Gain 1 : Gain  Gain=.5
  Product : Product
  Rear Wheel Angular Speed5 : Scope
      settings: YMin=0  YMax=2  SaveName=ScopeData5
  Sine Wave1 : Sin  Bias=1  Frequency=(pi/ck)  Phase=-pi/2  SampleTime=Ts
  Switch : Switch  Threshold=ck
  Output : Outport
  wires:
  Gain 1/1 -> Product/1, Rear Wheel Angular Speed5/1
  Sine Wave1/1 -> Switch/3
  Product/1 -> Output/1
  Input/1 -> Product/2
  Switch/1 -> Gain 1/1
  Digital Clock/1 -> Switch/2
  Constant1/1 -> Switch/1

== system conSys_3robots_1_vR2014a/Robot Space Controller/Clutch 7 ==
  Input : Inport
  Constant1 : Constant  Value=2
  Digital Clock : DigitalClock  SampleTime=Ts
  Gain 1 : Gain  Gain=.5
  Product : Product
  Rear Wheel Angular Speed5 : Scope
      settings: YMin=0  YMax=2  SaveName=ScopeData5
  Sine Wave1 : Sin  Bias=1  Frequency=(pi/ck)  Phase=-pi/2  SampleTime=Ts
  Switch : Switch  Threshold=ck
  Output : Outport
  wires:
  Constant1/1 -> Switch/1
  Digital Clock/1 -> Switch/2
  Switch/1 -> Gain 1/1
  Input/1 -> Product/2
  Product/1 -> Output/1
  Sine Wave1/1 -> Switch/3
  Gain 1/1 -> Rear Wheel Angular Speed5/1, Product/1

== system conSys_3robots_1_vR2014a/Robot Space Controller/Clutch 8 ==
  Input : Inport
  Constant1 : Constant  Value=2
  Digital Clock : DigitalClock  SampleTime=Ts
  Gain 1 : Gain  Gain=.5
  Product : Product
  Rear Wheel Angular Speed5 : Scope
      settings: YMin=0  YMax=2  SaveName=ScopeData5
  Sine Wave1 : Sin  Bias=1  Frequency=(pi/ck)  Phase=-pi/2  SampleTime=Ts
  Switch : Switch  Threshold=ck
  Output : Outport
  wires:
  Gain 1/1 -> Product/1, Rear Wheel Angular Speed5/1
  Sine Wave1/1 -> Switch/3
  Product/1 -> Output/1
  Input/1 -> Product/2
  Switch/1 -> Gain 1/1
  Digital Clock/1 -> Switch/2
  Constant1/1 -> Switch/1

== system conSys_3robots_1_vR2014a/Robot Space Controller/Clutch 9 ==
  Input : Inport
  Constant1 : Constant  Value=2
  Digital Clock : DigitalClock  SampleTime=Ts
  Gain 1 : Gain  Gain=.5
  Product : Product
  Rear Wheel Angular Speed5 : Scope
      settings: YMin=0  YMax=2  SaveName=ScopeData5
  Sine Wave1 : Sin  Bias=1  Frequency=(pi/ck)  Phase=-pi/2  SampleTime=Ts
  Switch : Switch  Threshold=ck
  Output : Outport
  wires:
  Constant1/1 -> Switch/1
  Digital Clock/1 -> Switch/2
  Switch/1 -> Gain 1/1
  Input/1 -> Product/2
  Product/1 -> Output/1
  Sine Wave1/1 -> Switch/3
  Gain 1/1 -> Rear Wheel Angular Speed5/1, Product/1

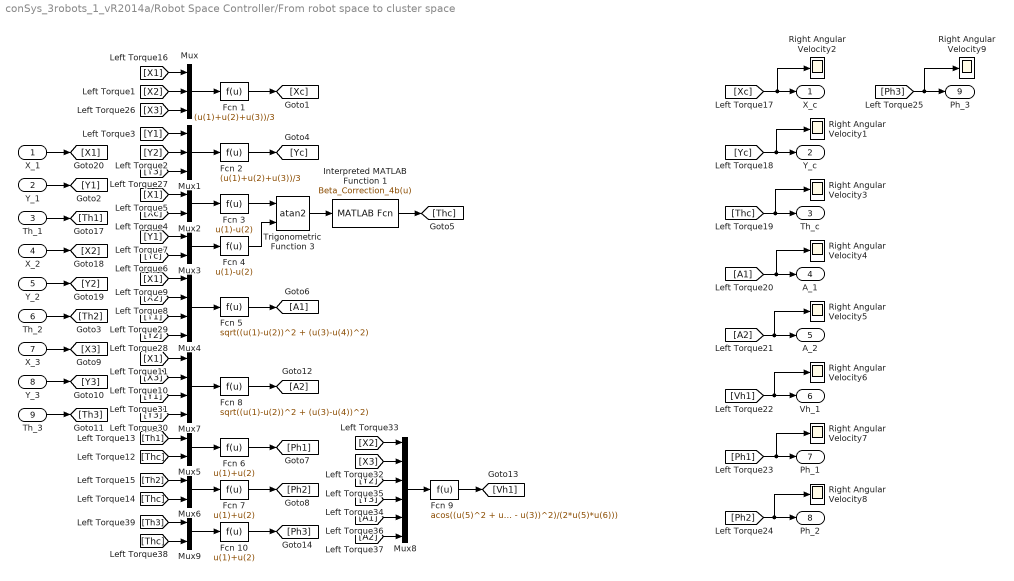
== system conSys_3robots_1_vR2014a/Robot Space Controller/From robot space to cluster space ==
  X_1 : Inport
  Y_1 : Inport  Port=2
  Th_1 : Inport  Port=3
  X_2 : Inport  Port=4
  Y_2 : Inport  Port=5
  Th_2 : Inport  Port=6
  X_3 : Inport  Port=7
  Y_3 : Inport  Port=8
  Th_3 : Inport  Port=9
  Fcn 1 : Fcn  Expr=(u(1)+u(2)+u(3))/3
  Fcn 10 : Fcn  Expr=u(1)+u(2)
  Fcn 2 : Fcn  Expr=(u(1)+u(2)+u(3))/3
  Fcn 3 : Fcn  Expr=u(1)-u(2)
  Fcn 4 : Fcn  Expr=u(1)-u(2)
  Fcn 5 : Fcn  Expr=sqrt((u(1)-u(2))^2 + (u(3)-u(4))^2)
  Fcn 6 : Fcn  Expr=u(1)+u(2)
  Fcn 7 : Fcn  Expr=u(1)+u(2)
  Fcn 8 : Fcn  Expr=sqrt((u(1)-u(2))^2 + (u(3)-u(4))^2)
  Fcn 9 : Fcn  Expr=acos((u(5)^2 + u(6)^2 - (u(2) - u(1))^2 - (u(4) - u(3))^2)/(2*u(5)*u(6)))
  Interpreted MATLAB Function 1 : MATLABFcn  MATLABFcn=Beta_Correction_4b(u)  SampleTime=Ts
  Mux : Mux  Inputs=3
  Mux1 : Mux  Inputs=3
  Mux{2..3,5..6,9} (5 alike) : Mux  Inputs=2
  Mux4 : Mux
  Mux7 : Mux
  Mux8 : Mux  Inputs=6
  Right Angular Velocity{1..9} (9 alike) : Scope
      Right Angular Velocity1 settings: YMin=2400  YMax=2600  SaveName=ScopeData38
      Right Angular Velocity2 settings: YMin=2400  YMax=2600  SaveName=ScopeData36
      Right Angular Velocity3 settings: YMin=-20  YMax=20  SaveName=ScopeData48
      Right Angular Velocity4 settings: YMin=0  YMax=1000  SaveName=ScopeData49
      Right Angular Velocity5 settings: YMin=0  YMax=1000  SaveName=ScopeData50
      Right Angular Velocity6 settings: SaveName=ScopeData51
      Right Angular Velocity7 settings: YMin=-20  YMax=20  SaveName=ScopeData87
      Right Angular Velocity8 settings: YMin=-20  YMax=20  SaveName=ScopeData88
      Right Angular Velocity9 settings: YMin=-20  YMax=20  SaveName=ScopeData89
  Trigonometric Function 3 : Trigonometry  Operator=atan2
  X_c : Outport
  Y_c : Outport  Port=2
  Th_c : Outport  Port=3
  A_1 : Outport  Port=4
  A_2 : Outport  Port=5
  Vh_1 : Outport  Port=6
  Ph_1 : Outport  Port=7
  Ph_2 : Outport  Port=8
  Ph_3 : Outport  Port=9
  wires:
  Y_2/1 -> [Y2]
  X_2/1 -> [X2]
  Th_1/1 -> [Th1]
  Y_1/1 -> [Y1]
  X_1/1 -> [X1]
  Th_2/1 -> [Th2]
  [X2] -> Mux/2
  [X1] -> Mux/1
  Mux/1 -> Fcn 1/1
  Fcn 1/1 -> [Xc]
  [Y2] -> Mux1/2
  [Y1] -> Mux1/1
  Mux1/1 -> Fcn 2/1
  Fcn 2/1 -> [Yc]
  [X1] -> Mux2/1
  [Yc] -> Mux3/2
  [Xc] -> Mux2/2
  [Y1] -> Mux3/1
  Interpreted MATLAB Function 1/1 -> [Thc]
  Trigonometric Function 3/1 -> Interpreted MATLAB Function 1/1
  Mux2/1 -> Fcn 3/1
  Mux3/1 -> Fcn 4/1
  Fcn 3/1 -> Trigonometric Function 3/1
  Fcn 4/1 -> Trigonometric Function 3/2
  [X1] -> Mux4/1
  [X2] -> Mux4/2
  Mux4/1 -> Fcn 5/1
  Fcn 5/1 -> [A1]
  [Th1] -> Mux5/1
  [Thc] -> Mux5/2
  Mux5/1 -> Fcn 6/1
  Fcn 6/1 -> [Ph1]
  [Th2] -> Mux6/1
  [Thc] -> Mux6/2
  Mux6/1 -> Fcn 7/1
  Fcn 7/1 -> [Ph2]
  [Xc] -> Right Angular Velocity2/1, X_c/1
  [Yc] -> Right Angular Velocity1/1, Y_c/1
  [Thc] -> Right Angular Velocity3/1, Th_c/1
  [A1] -> Right Angular Velocity4/1, A_1/1
  [A2] -> Right Angular Velocity5/1, A_2/1
  [Vh1] -> Right Angular Velocity6/1, Vh_1/1
  Y_3/1 -> [Y3]
  X_3/1 -> [X3]
  Th_3/1 -> [Th3]
  [Ph1] -> Ph_1/1, Right Angular Velocity7/1
  [Ph2] -> Ph_2/1, Right Angular Velocity8/1
  [Ph3] -> Ph_3/1, Right Angular Velocity9/1
  [X3] -> Mux/3
  [Y3] -> Mux1/3
  [Th3] -> Mux9/1
  [Thc] -> Mux9/2
  Mux9/1 -> Fcn 10/1
  Fcn 10/1 -> [Ph3]
  [X1] -> Mux7/1
  [X3] -> Mux7/2
  Mux7/1 -> Fcn 8/1
  Fcn 8/1 -> [A2]
  [Y2] -> Mux4/4
  [Y1] -> Mux4/3
  [Y1] -> Mux7/3
  [Y3] -> Mux7/4
  [X2] -> Mux8/1
  [X3] -> Mux8/2
  Mux8/1 -> Fcn 9/1
  Fcn 9/1 -> [Vh1]
  [Y2] -> Mux8/3
  [Y3] -> Mux8/4
  [A1] -> Mux8/5
  [A2] -> Mux8/6
